simulink model "Super10"  (Simulink 5.0)
settings: Solver=ode45  StartTime=0.0  StopTime=10.0  RelTol=1e-3
settings Model: Creator=scaife  LastModifiedBy=scaife  ExtModeAutoUpdateStatusClock=off

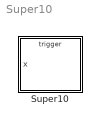
== system Super10 ==
  Super10 : Stateflow chart

== stateflow chart Super10 ==
  state A
  state B
    state B1
    state B2
    B1 -> B2 : E
    (default) -> B1
  (default) -> A
  A -> (junction 7) : E
  B2 -> A : E
  (junction 7) -> B : [x==0]
  (junction 7) -> B2 : [x<>0]
  data: x input int32
  events: E input EITHER_EDGE_EVENT
